simulink model "untitled"  (R2021b)
settings: Solver=FixedStepAuto  StartTime=0.0  StopTime=50  FixedStep=0.01  RelTol=1e-3
settings Model: Creator=osini  LastModifiedBy=osini

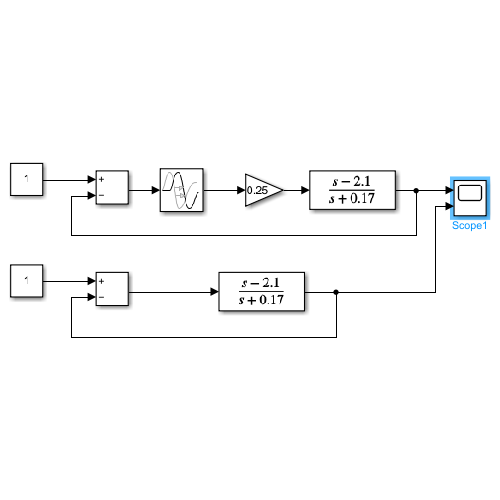
[thumbnail: Simulink's stored preview of the top-level diagram]
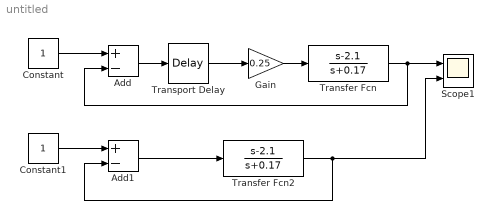
== system untitled ==
  Add : Sum  Inputs=+-
  Add1 : Sum  Inputs=+-
  Constant : Constant
  Constant1 : Constant
  Gain : Gain  Gain=0.25
  Scope1 : Scope  NumInputPorts=2
  Transfer Fcn : TransferFcn  Numerator=[1 -2.1]  Denominator=[1 0.17]
  Transfer Fcn2 : TransferFcn  Numerator=[1 -2.1]  Denominator=[1 0.17]
  Transport Delay : TransportDelay  InitialOutput=0.01
  wires:
  Constant/1 -> Add/1
  Add/1 -> Transport Delay/1
  Transport Delay/1 -> Gain/1
  Transfer Fcn/1 -> Scope1/1, Add/2
  Transfer Fcn2/1 -> Scope1/2, Add1/2
  Constant1/1 -> Add1/1
  Gain/1 -> Transfer Fcn/1
  Add1/1 -> Transfer Fcn2/1
